simulink model "simple_chart_demo"  (R2023a)
settings: Solver=VariableStepAuto  StartTime=0.0  StopTime=inf  RelTol=1e-3
settings Model: Creator=nkobayas  LastModifiedBy=nkobayas

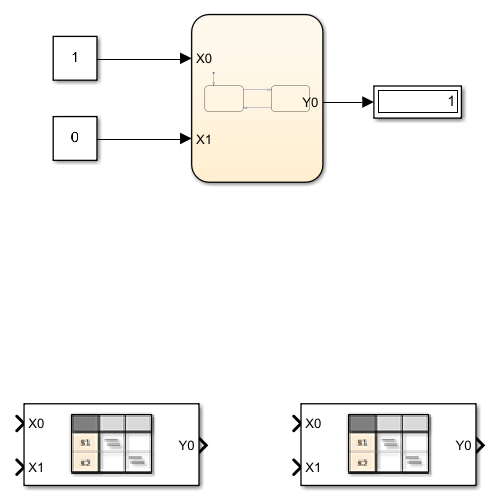
[thumbnail: Simulink's stored preview of the top-level diagram]
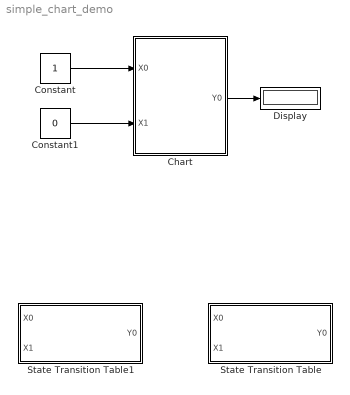
== system simple_chart_demo ==
  Chart : Stateflow chart  TreatAsAtomicUnit=on
  Constant : Constant
  Constant1 : Constant  Value=0
  Display : Display
  State Transition Table : State Transition Table  TreatAsAtomicUnit=on
  State Transition Table1 : State Transition Table  TreatAsAtomicUnit=on
  wires:
  Constant/1 -> Chart/1(X0)
  Constant1/1 -> Chart/2(X1)
  Chart/1(Y0) -> Display/1

== stateflow chart simple_chart_demo/State Transition Table1 ==
  state OFF
    Y0 = false;
  state ON
    Y0 = true;
  (default) -> OFF
  OFF -> ON : [X0]
  ON -> OFF : [X1]
  data: Y0 output; X0 input; X1 input

== stateflow chart simple_chart_demo/Chart ==
  state OFF
    Y0 = false;
  state ON
    Y0 = true;
  (default) -> OFF
  OFF -> ON : [(X0==true)&&...
      | (X1==false)]
  ON -> OFF : [(X1==true)&&...
      | (X0==false)]
  data: X0 input; X1 input; Y0 output

== stateflow chart simple_chart_demo/State Transition Table ==
  state OFF
    Y0 = false;
  state ON
    Y0 = true;
  (default) -> OFF
  OFF -> ON : [X0==true&&X1==false]
  ON -> OFF : [X0==true&&X1==false]
  data: Y0 output; X0 input; X1 input
